simulink model "robotracer_simulation_gazebo_simulink"  (R2020a)
settings: Solver=VariableStepAuto  StartTime=0.0  StopTime=5  RelTol=1e-3
undefined symbols (not defined in the file or in its folder): Angular, Linear
libraries: robotlib x3, robotgazebolib x2, simulink x2
settings Model: EnablePacing=on  Creator=under  LastModifiedBy=under

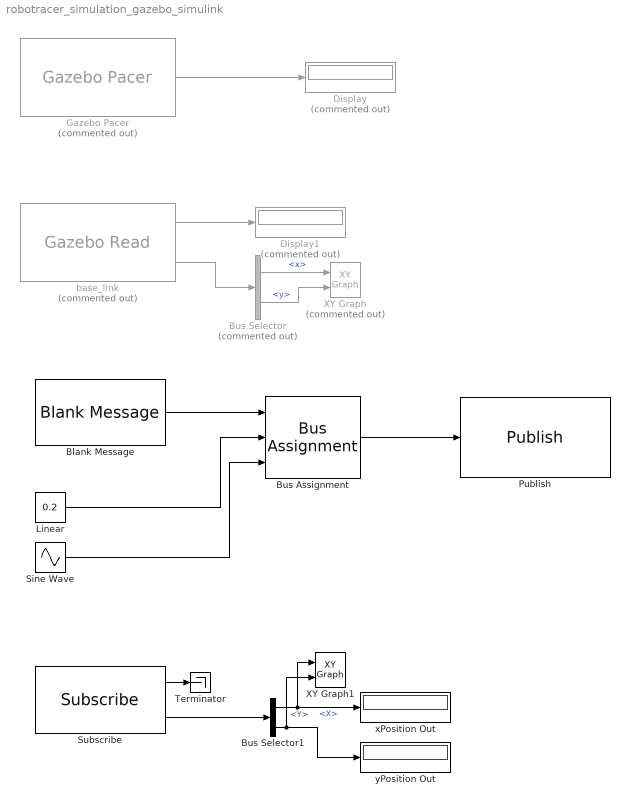
== system robotracer_simulation_gazebo_simulink ==
  Blank Message : robotlib/Blank Message  messageClass=Message  entityType=geometry_msgs/Twist  messageType=geometry_msgs/Twist  SampleTime=-1
  Bus Assignment : BusAssignment  AssignedSignals=Linear.X,Angular.Z
  Bus Selector : BusSelector  Commented=on  OutputSignals=position.x,position.y
  Bus Selector1 : BusSelector  DialogController=Simulink.DDGSource_BusSelector  OutputSignals=Pose.Pose.Position.X,Pose.Pose.Position.Y
  Display : Display  Commented=on
  Display1 : Display  Commented=on
  Gazebo Pacer : robotgazebolib/Gazebo Pacer  Commented=on  ResetBehavior=Reset Gazebo simulation time and scene  SampleTime=0.01
      settings: SourceProductBaseCode=RO
  Linear : Constant  Value=0.2
  Publish : robotlib/Publish  topicSource=Select from ROS network  topic=/cmd_vel  messageType=geometry_msgs/Twist  messageQueueLength=1
  Sine Wave : Sin  Amplitude=0.1  SampleTime=0
  Subscribe : robotlib/Subscribe  topicSource=Select from ROS network  topic=/odom  messageType=nav_msgs/Odometry  sampleTime=-1  messageQueueLength=1
  Terminator : Terminator
  XY Graph : simulink/Sinks/XY Graph  Commented=on  xmin=0  xmax=5  ymin=-1  ymax=1  st=-1
  XY Graph1 : simulink/Sinks/XY Graph  xmin=10  xmax=15  ymin=-35  ymax=-30  st=-1
  base_link : robotgazebolib/Gazebo Read  Commented=on  topicSource=From Gazebo  topic=/gazebo/ground_truth/world_pose/robotracer_v1/base_link  messageType=gazebo_msgs/Pose  sampleTime=0.1
      settings: SourceProductBaseCode=RO
  xPosition Out : Display
  yPosition Out : Display
  wires:
  Gazebo Pacer/1 -> Display/1
  base_link/1 -> Display1/1
  base_link/2 -> Bus Selector/1
  Bus Selector/1 -> XY Graph/1  "<x>"
  Bus Selector/2 -> XY Graph/2  "<y>"
  Blank Message/1 -> Bus Assignment/1
  Linear/1 -> Bus Assignment/2
  Bus Assignment/1 -> Publish/1
  Bus Selector1/1 -> XY Graph1/1, xPosition Out/1  "<X>"
  Bus Selector1/2 -> yPosition Out/1, XY Graph1/2  "<Y>"
  Subscribe/2 -> Bus Selector1/1
  Subscribe/1 -> Terminator/1
  Sine Wave/1 -> Bus Assignment/3
